simulink model "effect"  (R2018b)
settings: Solver=VariableStepAuto  StartTime=0.0  StopTime=10.0  RelTol=1e-3
undefined symbols (not defined in the file or in its folder): dfilt
libraries: dspsnks4 x1, dspvision x1, dsparch4 x1, dspsrcs4 x1
settings Model: Creator=Jason  LastModifiedBy=Jason
settings SFSimCC: SimUseLocalCustomCode=off
settings RTWCC: RTWUseLocalCustomCode=off
settings CodeAppCC: StateflowObjectComments=on

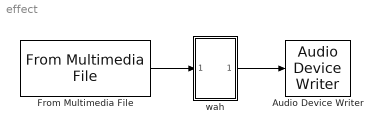
== system effect ==
  Audio Device Writer : dspsnks4/Audio Device Writer  Driver=DirectSound  Device=Default  InheritSampleRate=off  SampleRate=44100  BitDepth=16-bit integer  BufferSize=4096  NumBuffers=10  DefaultOutputChannelMapping=on  OutputChannelMapping=1:2  OutputNumUnderrunSamples=off  DriverIdx=1  DeviceWarnFlag=''
  From Multimedia File : dspvision/From Multimedia File  inputFilename=C:\Users\Jason\Desktop\Lab2\guitar1.wav  loop=on  numPlays=inf  outputStreams=Audio only  videoDataType=single  audioDataType=double  inheritSampleTime=on  userDefinedSampleTime=1/30  noAudioOutput=off  isIntensityVideo=off  fourcc=RGB  colorVideoFormat=Separate color signals  outputEOF=off  dataOrg=Column-major  audioFrameSize=1024  computeAudioFrameSize=off  outSamplingMode=Sample based
      settings: SourceProductBaseCode=VP
  wah : Subsystem
  wires:
  From Multimedia File/1 -> wah/1(In1)
  wah/1(Out1) -> Audio Device Writer/1

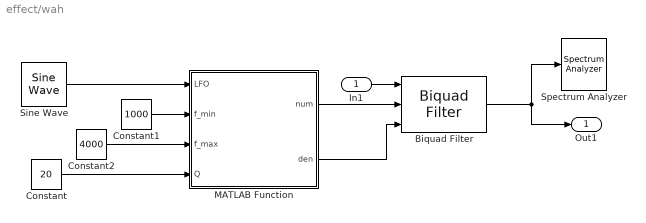
== system effect/wah ==
  In1 : Inport
  Biquad Filter : dsparch4/Biquad Filter  FilterSource=Input port(s)  CoeffSource=Specify via dialog  FilterObject=dfilt.df2tsos([1 0.3 0.4],[1 0.1 0.2])  IIRFiltStruct=Direct form II transposed  BiQuadCoeffs=[1 0.3 0.4 1 0.1 0.2]  ScaleValues=1  IC=0  ICnum=0  ICden=0  a0Flag=Warning  optimizeScaleValues=on  ScaleValueMode=Assume all are unity and optimize  InputProcessing=Columns as channels (frame based)  roundingMode=Floor  overflowMode=off  scaleValueFracLength=14  denProdOutputFracLength=30  denAccumFracLength=30  secondMemoryFracLength=15
      settings: SourceProductName=DSP System Toolbox
  Constant : Constant  Value=20
  Constant1 : Constant  Value=1000
  Constant2 : Constant  Value=4000
  MATLAB Function : MATLAB Function  TreatAsAtomicUnit=on
  Sine Wave : dspsrcs4/Sine Wave  Amplitude=1  Frequency=1  Phase=0  SampleMode=Discrete  OutComplex=Real  CompMethod=Trigonometric fcn  TableSize=Speed  SampleTime=1024/44100  SamplesPerFrame=1  ResetState=Restart at time zero  OutputFrames=off  dataType=double  wordLen=16  udDataType=sfix(16)  fracBitsMode=Best precision  numFracBits=15  OutDataTypeStr=double  LastOutDataTypeStr=double
  Spectrum Analyzer : SpectrumAnalyzer
  Out1 : Outport
  wires:
  In1/1 -> Biquad Filter/1
  MATLAB Function/1(num) -> Biquad Filter/2
  MATLAB Function/2(den) -> Biquad Filter/3
  Constant1/1 -> MATLAB Function/2(f_min)
  Constant2/1 -> MATLAB Function/3(f_max)
  Sine Wave/1 -> MATLAB Function/1(LFO)
  Constant/1 -> MATLAB Function/4(Q)
  Biquad Filter/1 -> Spectrum Analyzer/1, Out1/1

== matlab function effect/wah/MATLAB Function ==
  data: LFO input; num output; f_min input; f_max input; Q input; den output
function [num,den]  = iirNotchLFO(LFO, f_min, f_max, Q)
Fs = 44100;
f = 0.5*(f_max-f_min)*double(LFO)+(f_min+f_max)/2; % Shift/Scale Triangle wave
BW = pi*f/(Fs*Q);
Wo = f*pi/Fs;
gain = 1/(1+sqrt(1/2).*tan(BW/2));
num  = (1-gain)*[1 0 -1]';
den  = [-2*gain*cos(Wo) (2*gain-1)]';
end
